simulink model "LCC_TorqueControl_PID"  (R2023b)
settings: Solver=FixedStepAuto  StartTime=0.0  StopTime=10.0  FixedStep=simStepSize  RelTol=1e-3
libraries: dspstat3 x1
settings Model: Creator=balls  LastModifiedBy=scb548

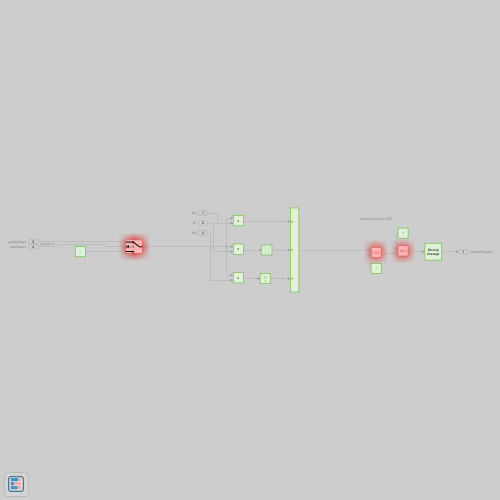
[thumbnail: Simulink's stored preview of the top-level diagram]
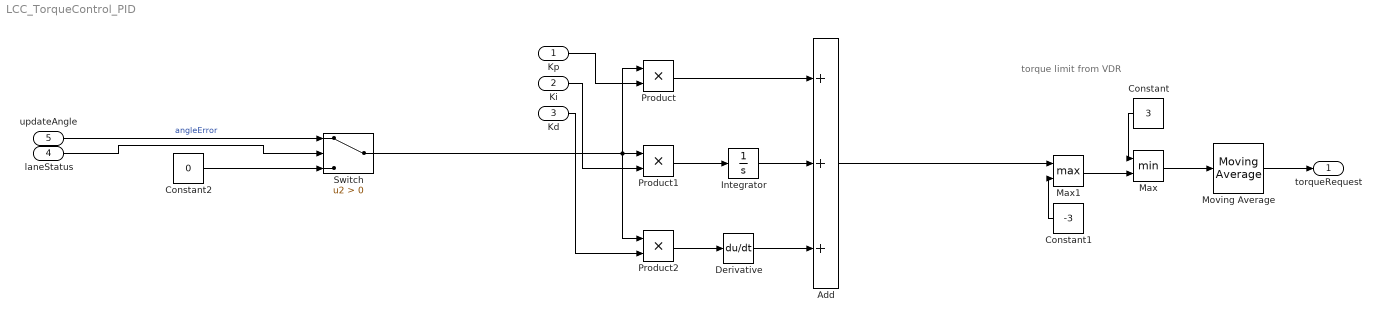
== system LCC_TorqueControl_PID ==
  note: torque limit from VDR
  Kp : Inport
  Ki : Inport  Port=2
  Kd : Inport  Port=3
  laneStatus : Inport  Port=4
  updateAngle : Inport  Port=5
  Add : Sum  Inputs=+++
  Constant : Constant  Value=3
  Constant1 : Constant  Value=-3
  Constant2 : Constant  Value=0
  Derivative : Derivative
  Integrator : Integrator  LimitOutput=on  UpperSaturationLimit=3  LowerSaturationLimit=-3
  Max : MinMax  Inputs=2
  Max1 : MinMax  Function=max  Inputs=2
  Moving Average : dspstat3/Moving Average  Method=Sliding window  ForgettingFactorPort=off  SpecifyWindowLength=on  WindowLength=3  OverlapLength=2  AllowArbitraryInputLength=off  ForgettingFactor=0.9  SimulateUsing=Code generation
  Product : Product
  Product1 : Product
  Product2 : Product
  Switch : Switch  Criteria=u2 > Threshold  SaturateOnIntegerOverflow=off  InputSameDT=off
  torqueRequest : Outport  OutMin=-3  OutMax=3
  wires:
  Constant/1 -> Max/1
  Product/1 -> Add/1
  Add/1 -> Max1/1
  Kp/1 -> Product/2
  Constant1/1 -> Max1/2
  Constant2/1 -> Switch/3
  Ki/1 -> Product1/2
  laneStatus/1 -> Switch/2
  Product2/1 -> Derivative/1
  Max1/1 -> Max/2
  Integrator/1 -> Add/2
  Product1/1 -> Integrator/1
  Kd/1 -> Product2/2
  Derivative/1 -> Add/3
  Switch/1 -> Product2/1, Product1/1, Product/1
  Max/1 -> Moving Average/1
  Moving Average/1 -> torqueRequest/1
  updateAngle/1 -> Switch/1  "angleError"
